simulink model "Estimationdataset1"  (R2023b)
settings: Solver=FixedStepAuto  StartTime=0.0  StopTime=60  FixedStep=1/4096  RelTol=1e-3
(part 2 of 2)

== matlab function Estimationdataset1/Stimulation Genarator/Enabled Subsystem/MATLAB Function ==
  data: Stimulation output
function Stimulation = Generator

Stimulation = [0	0	0	0	0	0	0	0	0	0	0	0	0	0	0	0	0	0	0	0	0	0	0	0	0
0	0	0	0	0	0	0	0	0	0	0	0	0	0	0	0	0	0	0	0	0	0	0	0	0
0	0	0	0	0	0	0	0	0	0	0	0	0	0	0	0	0	0	0	0	0	0	0	0	0
0	0	0	0	0	0	0	0	0	0	0	0	0	0	0	0	0	0	0	0	0	0	0	0	0
16.2614692746660	5.96809627713270	11.2804515687007	7.48167372261174	11.1710394068492	9.18371102232294	7.84375919868470	13.3395415222167	7.36731306862391	6.50268971969915	14.8890919531348	12.4076283500932	6.96292872282223	10.3114859854506	10.0471278881615	9.53082284018656	17.1980667045128	10.9947444552353	5.47202371438856	2.34150369423271	6.90160609975239	12.3008922644254	13.5613938598536	14.5824957038119	1.74931445822282
33.9956396922268	15.8114662916261	21.3653332761450	16.7661279685260	24.4662213132618	16.6113162955410	14.6191143496864	22.8019304219897	18.5058981721684	14.5725899813463	31.9706820794442	22.6818080753295	14.6778103071570	18.1622348098554	23.1727791802501	22.7155103553448	37.9117756556876	22.1590421871172	13.6231988938969	5.21470360200759	15.3951087524332	22.5436334841164	26.5272643877518	32.4069993599136	4.09151982211919
43.0407397349935	27.9747110759727	-24.0624661576345	25.5377658576773	16.9153118941055	21.0423056350282	23.1339427810230	36.5257935306664	23.9681509749386	19.2724977003084	45.5105956629466	28.6502957280079	16.2023401208902	22.8423879868633	32.8268041965304	37.7071961666090	-23.6907224801662	25.7118569705894	20.7628123747935	5.73602582224409	16.9822697603313	35.7519458643712	37.5365044835541	49.1381209867117	-0.138674965223259
-20656.6624406715	-1798.26357505405	-26298.5468043808	-6000.18779298503	-23595.4270986982	-18163.9802265052	-2283.51818031814	-16907.0410546585	-14633.7392639241	-13677.7252607443	-18400.9114314475	-6202.83727608965	-1621.16979214913	-2019.22948345943	-1312.86713919660	-7353.56694004176	-25955.9053352325	-16158.5270201694	-10219.6119748266	-10512.7481694267	-15052.3642705649	-15651.4576625775	-1461.31319425966	-4978.05538485248	-223.864865380240
-9874.65820312500	-34565.6171875000	612.364196777344	-31759.3125000000	-2201.17749023438	-11278.6005859375	-33230.8554687500	-13648.1796875000	-17623.7460937500	-19135.8300781250	-10897.5664062500	-29996.6230468750	-33075.3046875000	-33198.4726562500	-32771.0625000000	-28411.3984375000	3449.44775390625	-14739.9531250000	-24169.2265625000	-23616.3984375000	-17224.4277343750	-15473.1933593750	-32826.7421875000	-32445.2246093750	-28433.8339843750
16738.1933593750	18105.6171875000	12866.9785156250	23989.9257812500	13875.9160156250	18036.1835937500	20292.7871093750	19223.6523437500	20856.1562500000	21560.2070312500	18201.3144531250	24076.1542968750	18637.6894531250	19845.0996093750	17447.4394531250	24198.1835937500	11917.8447265625	20045.4023437500	23590.6582031250	23162.8535156250	21325.8164062500	20425.9531250000	18300.8476562500	24042.1406250000	7670.39306640625
-3313.55273437500	3845.34960937500	-2991.11328125000	-437.709045410156	-3136.37011718750	-3138.46704101563	2252.37963867188	-2952.32202148438	-2668.22045898438	-2697.90747070313	-3000.55786132813	-941.904724121094	3690.48315429688	2947.00097656250	4364.73242187500	-1398.76428222656	-3026.58618164063	-2689.89355468750	-2194.54956054688	-2457.57104492188	-2563.14697265625	-2768.12353515625	4006.21093750000	222.663940429688	9393.31835937500
-2103.41967773438	-2837.51806640625	-1700.56640625000	-2482.77172851563	-1585.21752929688	-1785.45996093750	-2586.60522460938	-1772.70019531250	-1800.83410644531	-1907.22534179688	-1719.10498046875	-2235.84399414063	-2591.71655273438	-2485.97094726563	-2622.95776367188	-2100.62304687500	-1489.69824218750	-1725.28393554688	-2087.50439453125	-2123.42431640625	-1873.41662597656	-1753.37817382813	-2655.40039062500	-2325.57055664063	-3017.45825195313
-1087.65209960938	-1487.24304199219	-837.685241699219	-1243.93225097656	-720.001281738281	-819.168334960938	-1166.07910156250	-797.215576171875	-804.233032226563	-861.290832519531	-768.099243164063	-994.881286621094	-1156.66381835938	-1083.35131835938	-1175.22631835938	-905.797790527344	-663.716552734375	-775.631286621094	-946.045959472656	-963.433959960938	-878.881958007813	-764.438171386719	-1196.25878906250	-1088.57275390625	-1404.88452148438
-544.403381347656	-752.565979003906	-371.473297119141	-618.349731445313	-294.224975585938	-360.656372070313	-532.310058593750	-341.688415527344	-336.110656738281	-376.404479980469	-313.492248535156	-446.105773925781	-515.059936523438	-471.238128662109	-525.102783203125	-388.060394287109	-246.762908935547	-319.127197265625	-420.606140136719	-440.011901855469	-395.715545654297	-312.577697753906	-532.624877929688	-497.072265625000	-638.107543945313
-209.803070068359	-328.277832031250	-82.1708679199219	-248.776489257813	-34.5771026611328	-77.1329040527344	-190.879898071289	-57.3911247253418	-58.8470191955566	-88.9773559570313	-42.6444244384766	-125.619560241699	-169.633483886719	-142.865142822266	-173.927474975586	-87.8222503662109	9.65015411376953	-47.2922439575195	-111.414566040039	-138.848693847656	-97.6393890380859	-49.9158973693848	-183.140319824219	-157.080596923828	-263.499359130859
-23.2132854461670	-75.7285156250000	77.1619186401367	-17.2723255157471	100.690826416016	71.9198989868164	14.7311363220215	101.106323242188	92.4556732177734	75.7505569458008	112.683959960938	64.3969497680664	40.1427612304688	55.4582290649414	41.6875152587891	93.3856811523438	141.353210449219	102.413940429688	64.7966918945313	36.3450469970703	72.9779510498047	105.924636840820	34.4559555053711	56.2911834716797	-32.3010177612305
57.7972640991211	58.3013153076172	138.094039916992	94.4524078369141	153.768005371094	135.853271484375	119.031463623047	168.892501831055	163.238540649414	156.357055664063	178.211257934570	146.332122802734	136.658081054688	159.801925659180	136.682220458984	171.522979736328	190.366378784180	164.008621215820	146.536972045898	117.737945556641	145.604766845703	171.966049194336	142.121444702148	161.162796020508	90.6373901367188
81.8368377685547	103.460800170898	145.906631469727	129.406326293945	162.494140625000	155.265777587891	150.980819702148	183.389175415039	173.461380004883	169.313720703125	184.949096679688	163.697494506836	163.583190917969	192.654983520508	171.616958618164	185.350189208984	195.768783569336	177.563964843750	170.387145996094	139.831817626953	164.531021118164	182.787292480469	171.025878906250	191.184432983398	132.554870605469
77.8965682983398	105.849426269531	136.427841186523	127.449630737305	141.480514526367	139.168014526367	144.350601196289	165.645141601563	160.463027954102	151.279602050781	164.616134643555	159.182449340820	158.528335571289	179.977264404297	173.900863647461	173.516723632813	181.131622314453	171.328918457031	166.927261352539	132.934204101563	152.887542724609	165.977218627930	174.200378417969	188.045379638672	135.632034301758
65.2655258178711	91.1077880859375	119.839248657227	111.202468872070	121.716430664063	123.249542236328	128.109558105469	142.220932006836	138.274765014648	133.575103759766	140.602066040039	142.216705322266	139.182998657227	165.638992309570	156.384414672852	152.173019409180	156.132675170898	144.882629394531	139.667068481445	113.177017211914	131.462310791016	149.236984252930	158.664505004883	167.284744262695	124.258453369141
56.9046249389648	80.7954406738281	97.4104309082031	95.6248321533203	106.301574707031	103.570953369141	109.948120117188	123.386138916016	117.335067749023	111.109405517578	126.528976440430	116.890136718750	117.837280273438	144.520919799805	128.008209228516	132.328826904297	140.573760986328	123.776885986328	115.745269775391	97.1794281005859	112.297454833984	127.315673828125	138.278518676758	145.774688720703	105.204757690430
50.1225051879883	70.4935073852539	95.6209259033203	81.8866806030273	102.746658325195	92.2425918579102	91.1261596679688	114.240402221680	108.426223754883	95.4948425292969	117.474029541016	105.024078369141	97.0712585449219	119.232589721680	115.000747680664	116.663909912109	138.384613037109	117.121124267578	103.844558715820	82.7714233398438	108.752334594727	117.184936523438	121.991806030273	133.614807128906	86.3107147216797
58.4611968994141	69.2811050415039	106.850555419922	87.0983886718750	119.321258544922	89.3425903320313	85.0743255615234	128.734893798828	112.636154174805	98.2588043212891	137.149185180664	105.516998291016	87.4943695068359	115.412658691406	109.003646850586	114.278884887695	154.235092163086	111.714187622070	110.162246704102	89.4043273925781	122.737152099609	128.013793945313	117.985015869141	139.583450317383	85.9660491943359
98.6989440917969	91.7978515625000	133.620803833008	114.040191650391	162.535125732422	117.023300170898	110.011398315430	163.028762817383	140.146453857422	128.252822875977	183.304458618164	131.149063110352	101.557769775391	132.643157958984	114.035537719727	149.973556518555	191.295135498047	134.968185424805	133.009796142578	126.696166992188	166.890502929688	159.801208496094	137.607818603516	178.041870117188	111.511550903320
138.026138305664	137.453887939453	165.400360107422	157.180816650391	204.498474121094	161.572799682617	160.008605957031	205.081924438477	183.525497436523	181.296157836914	226.028625488281	168.551208496094	139.350296020508	169.163284301758	138.116806030273	212.488113403320	239.045089721680	178.511001586914	175.577606201172	169.247589111328	218.804168701172	206.709228515625	183.800582885742	235.209869384766	158.765502929688
134.083661317901	165.573600802488	164.786212252524	188.858286582594	187.396516289017	179.009097373922	189.100955907586	209.011652903462	182.811367226747	211.392645429598	221.536535983330	185.158015886704	172.351989849264	191.616621330716	159.064420903019	228.092464231146	232.353775839074	193.607138370388	194.940931454408	171.273437585018	207.700436887970	210.305712168831	220.540943438270	249.531539186791	179.652885443640
97.8045967760335	146.225753601189	117.349479566767	152.996739225412	118.409670530228	139.425580834575	155.921329571106	148.810868621016	128.897888658361	170.320409074379	161.571287932783	151.196077005041	167.185364853355	177.985232339036	155.627375476491	163.743007692728	163.215035791311	157.720236397592	151.719229011384	121.183177992070	129.606279348214	163.108388174697	188.476418272932	198.021982446792	151.496636141054
35.7048783327083	79.0573484750653	57.5801327760869	88.9525257034274	54.5082658984635	64.6320644798548	87.3786093887541	78.6332063612781	69.5570411668054	91.2465752630354	90.3884045904227	83.3174456022953	107.723013416912	123.692633253824	107.397090517791	85.4809568071115	85.6347379862791	88.7805417077607	86.0725089122620	47.2953263755000	48.4335831188414	83.3212166465956	117.851722959037	112.492043800401	74.4194945127993
-13.9244982972534	4.58858142753660	11.0727978284122	24.9522948740578	9.72539278593127	5.18693759460384	16.7843780344484	23.3596611429922	26.7221873869857	30.5166720118670	31.7439119078631	30.6512811454219	41.7593080450005	55.0911352673948	64.6313259272231	26.2764571481559	36.6965632797625	32.8100376994364	31.0849673734116	-13.8179904412456	0.0388409165818055	30.3395965379487	45.5927320296187	43.5928457550087	7.35706433303455
-22.2608634151079	-15.1603676446282	-13.0784165430353	-9.03120925157738	-9.36964395826661	-13.4452848836922	-22.1953269815662	1.99294677500819	-5.24941064781977	-3.34253776612134	11.7029969226351	-0.0542465040006737	4.42748360538878	10.7228784888966	32.2146256975379	5.44535490792748	16.2404139318377	6.81083201500074	1.77401764299153	-24.1901207411392	-14.5622771658988	12.1953759016881	14.7950681377037	20.8409262661427	-16.5833557851611
-20.2118066745445	-22.8715415421705	-11.8401091563080	-16.3093071176451	-12.7975192938374	-14.9397674419507	-25.5591975680277	-5.11803382341720	-4.18079873914261	-9.73524724457361	9.21228040426892	-11.4612321673744	-7.97839230939937	-6.03939986792979	7.70664724865656	0.639355052896864	10.5886359086936	-2.25328852362257	-7.49652637503435	-28.1894553349846	-13.3037297209586	1.02434354919075	6.78290367261562	11.1711547296921	-26.2712271455607
-21.0556470861746	-24.0190060901031	-5.17731482641393	-13.6993419641052	-11.9412492765444	-9.35479101260658	-16.4984178917856	-0.122671512086062	-1.95790669601770	-5.27609417504871	8.27027534451565	-12.8872885853199	-12.4402018544225	-5.92670349410296	-3.63409637584862	2.19279350687864	13.3595598348200	-5.95048901301292	-7.58501285986193	-24.6318802794172	-8.06757877827931	3.81208296013933	3.49831831273822	11.4833680987611	-22.6410929889039
-20.9925084211049	-16.9422519450505	-1.65484722196324	-9.24095864728054	-4.45363101981383	-6.48898423978334	-11.5759946827159	5.19147684804852	0.415747883963005	-1.15115364137429	9.55437612823989	-5.19253517907497	-12.0776865671605	1.64551779221439	-8.72722435253714	7.52870045908783	15.0782237154269	-3.21712593588807	-2.52253468765043	-18.6426009544644	-0.586362664351068	8.58827999380947	2.55034999081043	10.8722464535921	-17.8775662261037
-13.5042550453211	-11.1870860676879	-2.81045249390455	-2.28857488734062	3.68402844849285	-2.83852884329678	-3.98043250344388	5.24943154785241	4.65535388505370	1.28074567177543	12.6384086578204	0.0190493845191487	-5.76617351274669	4.27396940500597	-3.59209028181863	7.90018142261127	15.3620512304218	-1.98405274208850	0.527594510286330	-11.6121678797191	4.42051531421518	10.2152315782407	5.26337661620176	12.6717198462985	-11.2070978411747
-3.61718619067773	-6.80171188998780	2.27672814340815	0.869150939288722	8.74415417126548	-1.23618094027816	0.656263805628191	9.40798590841742	7.61384664247307	2.67365020183065	12.2598559723773	5.49311534979099	-2.02793166066943	6.86985067247092	-1.57491453597719	9.93471811752063	17.3061952457380	3.66415616202858	1.09812115059656	-3.55091704803144	5.92759459756657	11.2749067435576	7.63299446818508	13.1098701759321	-2.29655963365225
2.04694320026859	-1.62744068225504	3.55208327246749	3.64250786738719	7.79654632535445	1.56285423243382	1.46026731473837	9.45640119364486	6.92897324263430	4.45188549192337	11.7952112796315	5.56053112531284	1.25305708820153	6.46047680041844	0.468312666191230	9.70374080385169	13.0012055773769	4.50716727248815	4.01322103404803	-0.369686058162882	7.19231622185922	9.74431753147078	7.52938776538713	10.9160004634346	-0.328085617445829
1.37934876607269	-0.349495508529335	2.32490944590505	2.19816007551398	4.11490531226493	1.84996355546180	1.78091548111908	4.85866661288509	3.32801759420293	2.99864919046699	5.96394020491192	2.77774176671994	1.77735351797906	3.51681493436534	0.776929755956725	5.09381771115907	5.89771610113285	2.50979994528497	2.96508515135879	-0.726834949013039	3.93809626839045	4.61445222132394	4.44141708081469	5.48624288975272	0.500465316701633
0	0	0	0	0	0	0	0	0	0	0	0	0	0	0	0	0	0	0	0	0	0	0	0	0
0	0	0	0	0	0	0	0	0	0	0	0	0	0	0	0	0	0	0	0	0	0	0	0	0
0	0	0	0	0	0	0	0	0	0	0	0	0	0	0	0	0	0	0	0	0	0	0	0	0
0	0	0	0	0	0	0	0	0	0	0	0	0	0	0	0	0	0	0	0	0	0	0	0	0
0	0	0	0	0	0	0	0	0	0	0	0	0	0	0	0	0	0	0	0	0	0	0	0	0];

== matlab function Estimationdataset1/Stimulation Genarator/MATLAB Function ==
  data: stimulation input; stimu input; point output; index input; index output
function [point,index] = Generator(stimulation,stimu,index)

if isempty(stimulation)
    stimulation = null;
end

if stimu == 1
    index = 1;
end

if index <length(stimulation)
    point = stimulation(index);
    index = index+1;
else
    point = 0;
end

== matlab function Estimationdataset1/Phase Estimation/State Space/Subsystem/MATLAB Function ==
  data: x input; y input; x_new output; P input; phi input; Q input; M input; P_new output; phase output; R input
function [x_new,P_new,phase] = Step(x,y,P,phi,Q,M,R)

x_one = phi *x;
P_one = phi *P * phi' + Q;

K_one = (P_one*M) /(M'*P_one*M + R); 

x_new = x_one + K_one * (y - M'*x_one);
P_new = P_one - K_one * M' * P_one;

P_new = (P_new + P_new') /2; % forcing symmetry to kill off rounding errors
phase = angle(x_new(1) + 1i* x_new(2));

== matlab function Estimationdataset1/Phase Estimation/Hilbert+AR/Hilbert+AR ==
  data: input input; phase output
function phase = fcn(input)
if length(input) >= 500

order = 24;
Hilbet_length = 128;
edge_length = 64;
iterations = edge_length + ceil(Hilbet_length/2);
data = input(edge_length+1:end-edge_length);

% AR model
estimated_coefficients = aryule(data, order);
coefficients = -1 * flip(estimated_coefficients(:, 2:end)');

% prepare matrix with the aditional time points for the forward prediction
data_filtered_withoutedge_predicted = [data', ones(1,iterations)];

% run the forward prediction
for i = iterations:-1:1
    %a = sum(coefficients .* data_filtered_withoutedge_predicted((end-i-order+1):(end-i))');
    data_filtered_withoutedge_predicted(end-i+1) = sum(coefficients .* data_filtered_withoutedge_predicted((end-i-order+1):(end-i))');
end

data_filtered_withoutedge_predicted_hilbertwindow = data_filtered_withoutedge_predicted(end-Hilbet_length+1:end);

% analytic signal and angle
data_filtered_withoutedge_predicted_hilbertwindow_analytic = hilbert(data_filtered_withoutedge_predicted_hilbertwindow);


phase = angle(data_filtered_withoutedge_predicted_hilbertwindow_analytic(end-iterations+edge_length));
%amplitude = mean(abs(data_filtered_withoutedge_predicted_hilbertwindow_analytic));

else
    phase = 0;
end
end

== matlab function Estimationdataset1/Phase Estimation/Zero-crossing/Zero-crossing ==
  data: input input; time input; phase_wrapped output; last input; out output; last_crossing input; frequency input; time output; instantaneous_frequency output; crossing output
function [phase_wrapped,out,time,instantaneous_frequency, crossing] = fcn(input,time,last,last_crossing,frequency)

fs = 4096;

if sign(input) ~= sign(last) && input>0
   T = (time - last_crossing)/fs;
   instantaneous_frequency = 1/T;
   frequency = instantaneous_frequency;
   crossing = time;
else
    crossing = last_crossing;
    instantaneous_frequency = frequency;
end


phase = -pi/2 + 2* pi * frequency * (time-crossing)/fs;
if phase>pi
    phase_wrapped = phase - 2*pi;
else
    phase_wrapped = phase;
end


out = input;
time = time+1;

== matlab function Estimationdataset1/Amplitude Estimation/Hilbert+AR1/Hilbert+AR ==
  data: input input; amp output
function amp = fcn(input)
if length(input) >= 500

order = 24;
Hilbet_length = 128;
edge_length = 64;
iterations = edge_length + ceil(Hilbet_length/2);
data = input(edge_length+1:end-edge_length);

% AR model
estimated_coefficients = aryule(data, order);
coefficients = -1 * flip(estimated_coefficients(:, 2:end)');

% prepare matrix with the aditional time points for the forward prediction
data_filtered_withoutedge_predicted = [data', ones(1,iterations)];

% run the forward prediction
for i = iterations:-1:1
    %a = sum(coefficients .* data_filtered_withoutedge_predicted((end-i-order+1):(end-i))');
    data_filtered_withoutedge_predicted(end-i+1) = sum(coefficients .* data_filtered_withoutedge_predicted((end-i-order+1):(end-i))');
end

data_filtered_withoutedge_predicted_hilbertwindow = data_filtered_withoutedge_predicted(end-Hilbet_length+1:end);

% analytic signal and angle
data_filtered_withoutedge_predicted_hilbertwindow_analytic = hilbert(data_filtered_withoutedge_predicted_hilbertwindow);

%amp = real(data_filtered_withoutedge_predicted_hilbertwindow_analytic(end-iterations+edge_length));
amp = abs(data_filtered_withoutedge_predicted_hilbertwindow_analytic(end-iterations+edge_length));

else
    amp = 0;
end
end

== matlab function Estimationdataset1/Pulse generator2/MATLAB Function1 ==
  data: input input; out output; previous input
function out  = fcn(input,previous)

Target = 3*pi/4;
if previous == 0
    if input >Target-0.02 && input < Target+0.02
        out = 1;
    else 
        out = 0;
    end
else
    out = 0;
end

end

== matlab function Estimationdataset1/Phase Estimation/State Space/MATLAB Function2 ==
  data: freq output; Fs output; ampVec output; sigmaFreqs output; sigmaObs output
function [freq,Fs,ampVec,sigmaFreqs,sigmaObs] = ini
freq = 21; 
Fs = 4096;
ampVec = 0.975;
sigmaFreqs = 1;
sigmaObs = 0.1;

== matlab function Estimationdataset1/Phase Estimation/State Space/MATLAB Function3 ==
  data: freq input; phi output; Fs input; ampVector input; sigmaFreqs input; Q output; M output
function [phi, Q, M] = genParametersSoulatMdl_sspp(freq, Fs,ampVector, sigmaFreqs)

    rotMat = zeros(2,2);
    varMat = zeros(2,2);

    rotMat(:,:) = [cos(2*pi*freq/Fs), -sin(2*pi*freq/Fs); ...
                  sin(2*pi*freq/Fs), cos(2*pi*freq/Fs)];
    rotMat(:,:) = rotMat(:,:) * ampVector;
    varMat( :,:) = [sigmaFreqs, 0; 0 , sigmaFreqs];


    phi = rotMat;
    Q = varMat;

    M = reshape([ones(1,1) , zeros(1,1)]', 1*2,1); % for extracting real part of signal from analytic 'x'


end

== matlab function Estimationdataset1/Phase Estimation/State Space/Subsystem/MATLAB Function4 ==
  data: sigmaObs input; x output; P output; R output
function [x,P,R] = fit_MKModel(sigmaObs)
% fitting the soulat model using the shumway-stoffer method (basically
% assuming no harmonics); EM has an analytic solution that needs the
% covariance structure between adjacent time points (this is what we need
% the fixed interval smoother for) 
% % This is the extension of the fitSoulatModel code to fit multiple
% sinusoids, still with no harmonics. 
% INPUTS:
% data - currently only accepts vector data so n x 1
% freqs - initialize with some frequencies that are appropriate for data
% Fs - sampling frequency
% sigmaFreqs - what are variances at each of the frequencies specified
% sibmaObs - what is the expected observation noise variance?
% Ani Wodeyar 3/17/2020
% have now fixed the indexing of the fixed interval smoother, was off by 1
% before
% Ani Wodeyar 9/23/2020

if isempty(sigmaObs)
    sigmaObs = 10;
end


% need to initialize all my parameters

R = sigmaObs;

stateVec = zeros(2,1);
stateCov = eye(2,2)*0.001;

x = stateVec(:,end);
P = squeeze(stateCov(:,:,end));

end

== matlab function Estimationdataset1/Amplitude Estimation/Non-Resonant Filter1/Subsystem/MATLAB Function ==
  data: x input; x output; xd input; alpha input; eta input; eetaDel input; ealDel input; C1 input; C2 input; C3 input; sprev input; s input; snew input; xd output
function [x,xd]=OneStep(x,xd,alpha,eta,eetaDel,ealDel,C1,C2,C3,sprev,s,snew) 
if isempty(x)
    x = 0;
end
if isempty(xd)
    xd = 0;
end
A=x-1i*(xd+alpha*x)/eta;
A=A-1i*(C1*sprev+C2*s+C3*snew)/eta;
d=A*eetaDel;
y=real(d); yd=real(1i*eta*(d-conj(d))/2);
x=y/ealDel; 
xd=(yd-alpha*y)/ealDel;
end

== matlab function Estimationdataset1/Amplitude Estimation/Non-Resonant Filter1/Subsystem/MATLAB Function1 ==
  data: om0 input; C1 output; alpha input; C2 output; C3 output; eetadel output; ealdel output; eta output
function [C1,C2,C3,eetadel,ealdel,eta]=ExSolCoefs(om0,alpha) 
% del is the time step dt
% alpha is the half of the dampling: x''+2*alpha*x'...
%fs = 20;
del = 1/4096;
eta2=om0^2-alpha^2; eta=sqrt(eta2);
eetadel=exp(1i*eta*del); a=1/eetadel; ealdel=exp(alpha*del);
I1=1i*(a-1)/eta; I2=(a*(1+1i*eta*del)-1)/eta2;
I3=(a*(del*eta*(2+1i*del*eta)-2*1i)+2*1i)/eta2/eta;
C1=(I3-I2*del)/2/del^2/ealdel;   C2=I1-I3/del^2;
C3=ealdel*(I2*del+I3)/2/del^2;
end

== matlab function Estimationdataset1/Amplitude Estimation/Non-Resonant Filter1/Subsystem/MATLAB Function3 ==
  data: x input; y input; Damp output; nu input; factor input
function Damp = AMP(x,y,nu,factor)
 z=y/nu;  Damp=factor*sqrt(z*z+x*x); % new amplitude value

== matlab function Estimationdataset1/Amplitude Estimation/Non-Resonant Filter1/Subsystem2/MATLAB Function2 ==
  data: om0 output; gama output; gamp output; nu output; factor output
function [om0, gama, gamp, nu, factor] = Initial
nu=2*pi*22;     % initial guess for frequency (10% large than the true value)
% parameters of the non-resonant "device"
om0=5*nu;  om0_2=om0*om0;         % oscillator frequency
alpha_a=80; gama=alpha_a/2;       % damping for the "amplitude device"     
alpha_p=10;  gamp=alpha_p/2;       % damping for the "phase device"
factor=sqrt((om0_2-nu*nu)^2+(alpha_a*nu)^2);

== matlab function Estimationdataset1/Amplitude Estimation/State Space1/MATLAB Function2 ==
  data: freq output; Fs output; ampVec output; sigmaFreqs output; sigmaObs output
function [freq,Fs,ampVec,sigmaFreqs,sigmaObs] = ini
freq = 21; 
Fs = 4096;
ampVec = 0.975;
sigmaFreqs = 1;
sigmaObs = 0.1;

== matlab function Estimationdataset1/Amplitude Estimation/State Space1/MATLAB Function3 ==
  data: freq input; phi output; Fs input; ampVector input; sigmaFreqs input; Q output; M output
function [phi, Q, M] = genParametersSoulatMdl_sspp(freq, Fs,ampVector, sigmaFreqs)

    rotMat = zeros(2,2);
    varMat = zeros(2,2);

    rotMat(:,:) = [cos(2*pi*freq/Fs), -sin(2*pi*freq/Fs); ...
                  sin(2*pi*freq/Fs), cos(2*pi*freq/Fs)];
    rotMat(:,:) = rotMat(:,:) * ampVector;
    varMat( :,:) = [sigmaFreqs, 0; 0 , sigmaFreqs];


    phi = rotMat;
    Q = varMat;

    M = reshape([ones(1,1) , zeros(1,1)]', 1*2,1); % for extracting real part of signal from analytic 'x'


end

== matlab function Estimationdataset1/Amplitude Estimation/State Space1/Subsystem/MATLAB Function ==
  data: x input; y input; x_new output; P input; phi input; Q input; M input; P_new output; amp output; R input
function [x_new,P_new,amp] = Step(x,y,P,phi,Q,M,R)

x_one = phi *x;
P_one = phi *P * phi' + Q;

K_one = (P_one*M) /(M'*P_one*M + R); 

x_new = x_one + K_one * (y - M'*x_one);
P_new = P_one - K_one * M' * P_one;

P_new = (P_new + P_new') /2; % forcing symmetry to kill off rounding errors
amp = abs(x_new(1) + 1i* x_new(2));

== matlab function Estimationdataset1/Amplitude Estimation/State Space1/Subsystem/MATLAB Function4 ==
  data: sigmaObs input; x output; P output; R output
function [x,P,R] = fit_MKModel(sigmaObs)
% fitting the soulat model using the shumway-stoffer method (basically
% assuming no harmonics); EM has an analytic solution that needs the
% covariance structure between adjacent time points (this is what we need
% the fixed interval smoother for) 
% % This is the extension of the fitSoulatModel code to fit multiple
% sinusoids, still with no harmonics. 
% INPUTS:
% data - currently only accepts vector data so n x 1
% freqs - initialize with some frequencies that are appropriate for data
% Fs - sampling frequency
% sigmaFreqs - what are variances at each of the frequencies specified
% sibmaObs - what is the expected observation noise variance?
% Ani Wodeyar 3/17/2020
% have now fixed the indexing of the fixed interval smoother, was off by 1
% before
% Ani Wodeyar 9/23/2020

if isempty(sigmaObs)
    sigmaObs = 10;
end


% need to initialize all my parameters

R = sigmaObs;

stateVec = zeros(2,1);
stateCov = eye(2,2)*0.001;

x = stateVec(:,end);
P = squeeze(stateCov(:,:,end));

end

== matlab function Estimationdataset1/Amplitude Estimation/Moving window/MATLAB Function ==
  data: input input; amp output
function amp = fcn(input)

amp = mean(abs(input(:)));

== matlab function Estimationdataset1/Phase Estimation/Non-Resonant Filter/Subsystem2/MATLAB Function2 ==
  data: om0 output; gama output; gamp output; nu output; factor output
function [om0, gama, gamp, nu, factor] = Initial
nu=2*pi*22;     % initial guess for frequency (10% large than the true value)
% parameters of the non-resonant "device"
om0=5*nu;  om0_2=om0*om0;         % oscillator frequency
alpha_a=80; gama=alpha_a/2;       % damping for the "amplitude device"     
alpha_p=10;  gamp=alpha_p/2;       % damping for the "phase device"
factor=sqrt((om0_2-nu*nu)^2+(alpha_a*nu)^2);

== matlab function Estimationdataset1/Phase Estimation/Non-Resonant Filter/Subsystem1/MATLAB Function4 ==
  data: om0 input; C1 output; alpha input; C2 output; C3 output; eetadel output; ealdel output; eta output
function [C1,C2,C3,eetadel,ealdel,eta]=ExSolCoefs(om0,alpha) 
% del is the time step dt
% alpha is the half of the dampling: x''+2*alpha*x'...
% fs = 20;
del = 1/4096;
eta2=om0^2-alpha^2; eta=sqrt(eta2);
eetadel=exp(1i*eta*del); a=1/eetadel; ealdel=exp(alpha*del);
I1=1i*(a-1)/eta; I2=(a*(1+1i*eta*del)-1)/eta2;
I3=(a*(del*eta*(2+1i*del*eta)-2*1i)+2*1i)/eta2/eta;
C1=(I3-I2*del)/2/del^2/ealdel;   C2=I1-I3/del^2;
C3=ealdel*(I2*del+I3)/2/del^2;
end

== matlab function Estimationdataset1/Phase Estimation/Non-Resonant Filter/Subsystem1/MATLAB Function5 ==
  data: x input; x output; xd input; alpha input; eta input; eetaDel input; ealDel input; C1 input; C2 input; C3 input; sprev input; s input; snew input; xd output
function [x,xd]=OneStep(x,xd,alpha,eta,eetaDel,ealDel,C1,C2,C3,sprev,s,snew) 
if isempty(x)
    x = 0;
end
if isempty(xd)
    xd = 0;
end
A=x-1i*(xd+alpha*x)/eta;
A=A-1i*(C1*sprev+C2*s+C3*snew)/eta;
d=A*eetaDel;
y=real(d); yd=real(1i*eta*(d-conj(d))/2);
x=y/ealDel; 
xd=(yd-alpha*y)/ealDel;
end

== matlab function Estimationdataset1/Phase Estimation/Non-Resonant Filter/Subsystem1/MATLAB Function6 ==
  data: u input; v input; Dphase output; nu input
function Dphase = PHA(u,v,nu)
 z = v/nu;  Dphase=atan2(-z,u);

== matlab function Estimationdataset1/Kalman filter/MATLAB Function ==
  data: A output; B output; H output; Qe output; Qt output; R output; width output
function [A,B,H,Qe,Qt,R,width]  = intitial

% Define Kalman filter model
% AR model estimation
%p = 2;
%a = arburg([xprev2,xprev1,x],p);
%A = [- a(2:(p+1)); eye(p-1, p)];
A = [1.9979830,-0.99963582;1,0];
B = [1; 0];
H = [1, 0];

% Setup for all the Kalman variables
% Noise matrices
sigmaE = 0.025;
sigmaT = 0.1;
sigmaV = 0.25;

% Initialize Q with initial values
Qe = diag([sigmaE, sigmaE]);
Qt = diag([sigmaE, sigmaT]);
R = sigmaV*60000000;% Set a high value so that artifact will not be trusted

fs = 4096;
width = floor(12*10^-3*fs);
